simulink library "nonentgaincalc"  (R2022b)
settings: Solver=VariableStepAuto  StartTime=0.0  StopTime=10.0  RelTol=1e-3
undefined symbols (not defined in the file or in its folder): boostOverRide, boostOverRideFlag, Fs, L, maxBoost, maxSPL, minVNCSignal, NoiseOverRide, NoiseOverRideFlag, VNCSlope, VNCThresh
libraries: NonEntGainCalcBtc x1
settings Model: Creator=ms51507  LastModifiedBy=kl13806
settings SolverCC: AlgebraicLoopSolver=TrustRegion
settings DebuggingCC: UnconnectedInputMsg=warning  UnconnectedOutputMsg=warning  UnconnectedLineMsg=warning  SFMachineParentedDataDiag=warning
settings ModelReferenceCC: EnableRefExpFcnMdlSchedulingChecks=on
settings RTWCC: DLArmComputeVersion=19.05

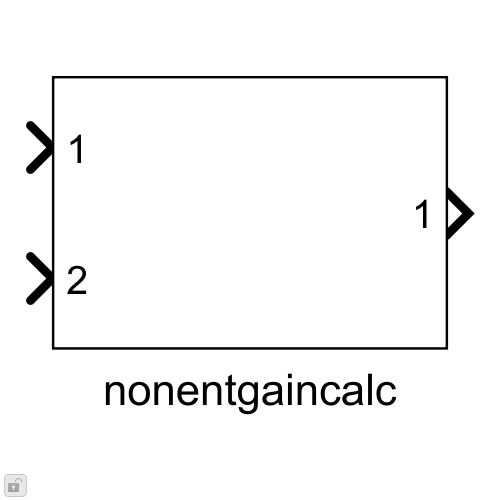
[thumbnail: Simulink's stored preview of the top-level diagram]
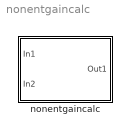
== system nonentgaincalc ==
  nonentgaincalc : Subsystem  mask(Bose nonentgaincalc){VNCThresh=VNCThresh, VNCSlope=VNCSlope, maxBoost=maxBoost, maxSPL=maxSPL, minVNCSignal=minVNCSignal, rampCoef=0, Fd=Fs/L, L=L, NoiseOverRideFlag=NoiseOverRideFlag, NoiseOverRide=NoiseOverRide, boostOverRideFlag=boostOverRideFlag, boostOverRide=boostOverRide}
      mask prompts: VNCThresh "VNC Threshold"; VNCSlope "VNC Slope"; maxBoost "Max Boost"; maxSPL "Max SPL"; minVNCSignal "Min VNC Signal"; rampCoef "Ramp Coefficients"; Fd "Decimated Rate (Fd)"; L "Frame Size"; NoiseOverRideFlag "Noise OverRide Flag"; NoiseOverRide "Noise OverRide Value"; boostOverRideFlag "Boost OverRide Flag"; boostOverRide "Boost OverRide Value"
      mask init:
      | blkh = gcbh;
      | % Copy discrete mask parameters into a classdef object
      | InnerLinkConfig = NonEntGainCalcConfig;
      | InnerLinkConfig.DefaultVncThresh = VNCThresh;
      | InnerLinkConfig.DefaultVncSlope = VNCSlope;
      | InnerLinkConfig.DefaultMaxBoost = maxBoost;
      | InnerLinkConfig.DefaultMaxSpl = maxSPL;
      | InnerLinkConfig.DefaultMinVncSignal = minVNCSignal;
      | InnerLinkConfig.RampCoef = rampCoef;
      | InnerLinkConfig.Fd = Fd;
      | InnerLinkConfig.FrameSize = L;
      | InnerLinkConfig.DefaultNoiseOverrideFlag = NoiseOverRideFlag;
      | InnerLinkConfig.DefaultNoiseOverride = NoiseOverRide;
      | InnerLinkConfig.DefaultBoostOverrideFlag = boostOverRideFlag;
      | InnerLinkConfig.DefaultBoostOverride = boostOverRide;
      mask DialogControl ParameterGroupVar2 Prompt: OverRides

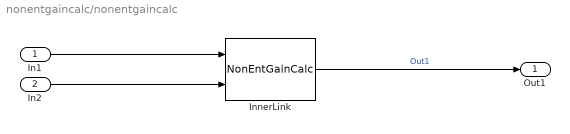
== system nonentgaincalc/nonentgaincalc ==
  In1 : Inport
  In2 : Inport  Port=2
  InnerLink : NonEntGainCalcBtc/NonEntGainCalc  Config=InnerLinkConfig  FeatureName=GainCalc
      settings: SourceProductName=Bose Blocklib
  Out1 : Outport
  wires:
  InnerLink/1 -> Out1/1  "Out1"
  In1/1 -> InnerLink/1
  In2/1 -> InnerLink/2
